simulink model "BitwiseOR_uint8"  (R2017b)
settings: Solver=ode3  StartTime=0.0  StopTime=10.0  FixedStep=0.200000  RelTol=1e-3
libraries: simulink x3
settings Model: Creator=hbourbou  LastModifiedBy=hbourbou
settings OptimizationCC: LifeSpan=inf
settings DebuggingCC: SFExecutionAtInitializationDiag=none
settings HardwareCC: ProdBitPerSizeT=32  ProdBitPerPtrDiffT=32  ProdWordSize=32  ProdHWDeviceType=Specified
settings CodeAppCC: StateflowObjectComments=on

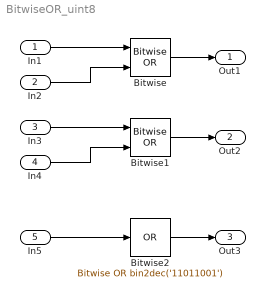
== system BitwiseOR_uint8 ==
  In1 : Inport  OutDataTypeStr=uint8
  In2 : Inport  Port=2  OutDataTypeStr=uint8
  In3 : Inport  Port=3  OutDataTypeStr=uint8
  In4 : Inport  Port=4  OutDataTypeStr=uint8  PortDimensions=3
  In5 : Inport  Port=5  OutDataTypeStr=uint8  PortDimensions=3
  Bitwise : simulink/Logic and Bit Operations/Bitwise Operator  logicop=OR  UseBitMask=off  NumInputPorts=2  BitMask=bin2dec('11011001')  BitMaskRealWorld=Stored Integer
  Bitwise1 : simulink/Logic and Bit Operations/Bitwise Operator  logicop=OR  UseBitMask=off  NumInputPorts=2  BitMask=bin2dec('11011001')  BitMaskRealWorld=Stored Integer
  Bitwise2 : simulink/Logic and Bit Operations/Bitwise Operator  logicop=OR  UseBitMask=on  BitMask=bin2dec('11011001')  BitMaskRealWorld=Stored Integer
  Out1 : Outport
  Out2 : Outport  Port=2
  Out3 : Outport  Port=3
  wires:
  In1/1 -> Bitwise/1
  In2/1 -> Bitwise/2
  Bitwise/1 -> Out1/1
  Bitwise1/1 -> Out2/1
  In3/1 -> Bitwise1/1
  In4/1 -> Bitwise1/2
  In5/1 -> Bitwise2/1
  Bitwise2/1 -> Out3/1
